simulink model "plant898708"  (R2016b)
settings: Solver=VariableStepAuto  StartTime=0.0  StopTime=800  RelTol=0.6
InitFcn:
  | data898708
undefined symbols (not defined in the file): En, ien, J, Keq, ki_ie, ki_ome, kp_ia, kp_ie, kp_ome, kr, La, Le, M, ome_n, r, Ra, Re, Ti_ia, Ti_ie, Ti_ome
settings Model: Creator=caidomenico  LastModifiedBy=caidomenico
settings SolverCC: ZeroCrossAlgorithm=Adaptive

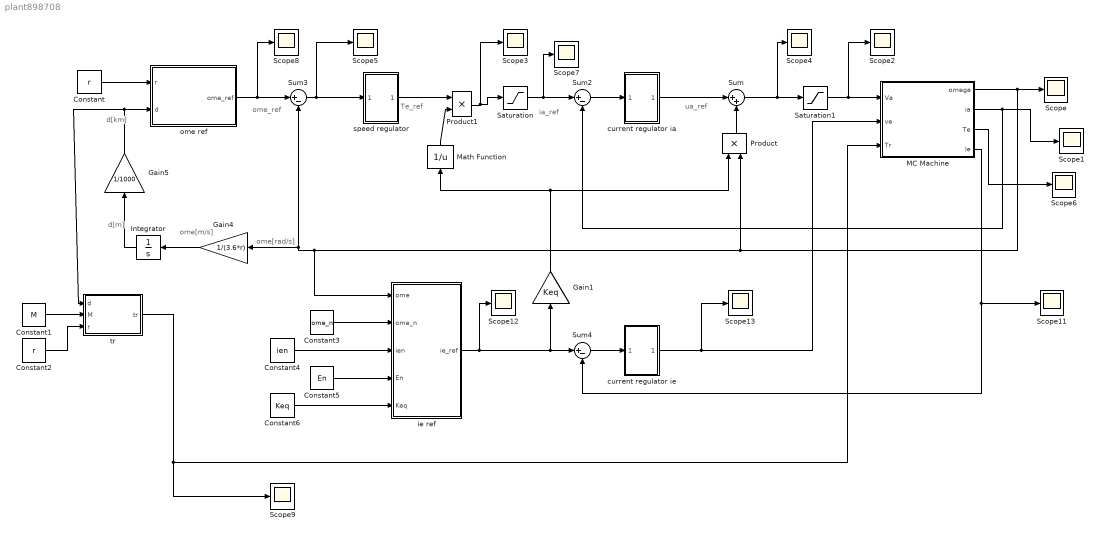
== system plant898708 ==
  note: ua_ref
  note: ia_ref
  note: Te_ref
  note: ome_ref
  note: d[km]
  note: d[m]
  note: ome[rad/s]
  note: ome[m/s]
  Constant : Constant  Value=r
  Constant1 : Constant  Value=M
  Constant2 : Constant  Value=r
  Constant3 : Constant  Value=ome_n
  Constant4 : Constant  Value=ien
  Constant5 : Constant  Value=En
  Constant6 : Constant  Value=Keq
  Gain1 : Gain  Gain=Keq
  Gain4 : Gain  Gain=1/(3.6*r)
  Gain5 : Gain  Gain=1/1000
  Integrator : Integrator
  MC Machine : Subsystem
      mask DialogControl DescTextVar Prompt: %<DC>
  Math Function : Math  Operator=reciprocal  SaturateOnIntegerOverflow=on
  Product : Product
  Product1 : Product
  Saturation : Saturate  UpperLimit=713  LowerLimit=0
  Saturation1 : Saturate  UpperLimit=600
  Scope{,1..9,11..13} (13 alike) : Scope
  Sum : Sum  Inputs=|++
  Sum2 : Sum  Inputs=|+-
  Sum3 : Sum  Inputs=|+-
  Sum4 : Sum  Inputs=|+-
  current regulator ia : Subsystem
  current regulator ie : Subsystem
  ie ref : MATLAB Function  TreatAsAtomicUnit=on
  ome ref : MATLAB Function  TreatAsAtomicUnit=on
  speed regulator : Subsystem
  tr : MATLAB Function  TreatAsAtomicUnit=on
  wires:
  Sum3/1 -> speed regulator/1(In1), Scope5/1
  MC Machine/1(omega) -> Product/2, ie ref/1(ome), Sum3/2, Gain4/1, Scope/1
  MC Machine/2(ia) -> Sum2/2, Scope1/1
  Sum/1 -> Scope4/1, Saturation1/1
  Saturation1/1 -> Scope2/1, MC Machine/1(Va)
  MC Machine/3(Te) -> Scope6/1
  ome ref/1(ome_ref) -> Scope8/1, Sum3/1
  Gain4/1 -> Integrator/1
  Integrator/1 -> Gain5/1
  Gain5/1 -> tr/1(d), ome ref/2(d)
  Constant/1 -> ome ref/1(r)
  speed regulator/1(Out1) -> Product1/1
  Constant3/1 -> ie ref/2(ome_n)
  Constant4/1 -> ie ref/3(ien)
  Constant5/1 -> ie ref/4(En)
  Constant6/1 -> ie ref/5(Keq)
  ie ref/1(ie_ref) -> Sum4/1, Gain1/1, Scope12/1
  Sum4/1 -> current regulator ie/1(In1)
  MC Machine/4(le) -> Scope11/1, Sum4/2
  current regulator ie/1(Out1) -> Scope13/1, MC Machine/2(ve)
  Sum2/1 -> current regulator ia/1(In1)
  current regulator ia/1(Out1) -> Sum/1
  Product1/1 -> Saturation/1, Scope3/1
  Product/1 -> Sum/2
  Gain1/1 -> Product/1, Math Function/1
  Math Function/1 -> Product1/2
  Saturation/1 -> Scope7/1, Sum2/1
  Constant1/1 -> tr/2(M)
  tr/1(tr) -> Scope9/1, MC Machine/3(Tr)
  Constant2/1 -> tr/3(r)

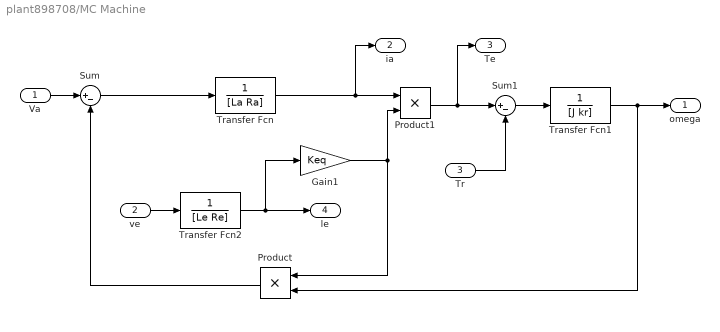
== system plant898708/MC Machine ==
  Va : Inport
  ve : Inport  Port=2
  Tr : Inport  Port=3
  Gain1 : Gain  Gain=Keq
  Product : Product
  Product1 : Product
  Sum : Sum  Inputs=|+-
  Sum1 : Sum  Inputs=|+-
  Transfer Fcn : TransferFcn  Denominator=[La Ra]
  Transfer Fcn1 : TransferFcn  Denominator=[J kr]
  Transfer Fcn2 : TransferFcn  Denominator=[Le Re]
  omega : Outport
  ia : Outport  Port=2
  Te : Outport  Port=3
  le : Outport  Port=4
  wires:
  Va/1 -> Sum/1
  Transfer Fcn/1 -> Product1/1, ia/1
  Sum/1 -> Transfer Fcn/1
  Transfer Fcn1/1 -> omega/1, Product/2
  ve/1 -> Transfer Fcn2/1
  Transfer Fcn2/1 -> le/1, Gain1/1
  Product1/1 -> Te/1, Sum1/1
  Gain1/1 -> Product/1, Product1/2
  Product/1 -> Sum/2
  Tr/1 -> Sum1/2
  Sum1/1 -> Transfer Fcn1/1

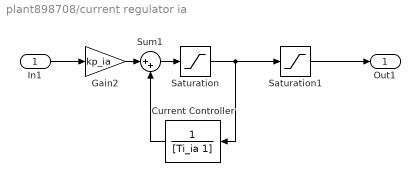
== system plant898708/current regulator ia ==
  In1 : Inport
  Current Controller : TransferFcn  Denominator=[Ti_ia 1]
  Gain2 : Gain  Gain=kp_ia
  Saturation : Saturate  UpperLimit=600
  Saturation1 : Saturate  UpperLimit=600
  Sum1 : Sum  Inputs=|++
  Out1 : Outport
  wires:
  Gain2/1 -> Sum1/1
  In1/1 -> Gain2/1
  Current Controller/1 -> Sum1/2
  Sum1/1 -> Saturation/1
  Saturation/1 -> Saturation1/1, Current Controller/1
  Saturation1/1 -> Out1/1

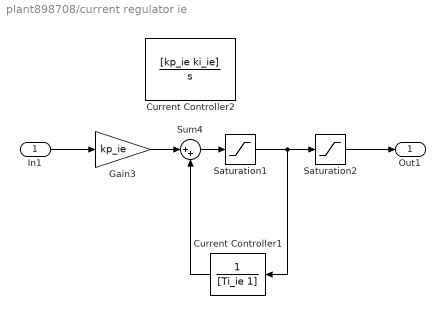
== system plant898708/current regulator ie ==
  In1 : Inport
  Current Controller1 : TransferFcn  Denominator=[Ti_ie 1]
  Current Controller2 : TransferFcn  Numerator=[kp_ie ki_ie]  Denominator=[1 0]
  Gain3 : Gain  Gain=kp_ie
  Saturation1 : Saturate  UpperLimit=120  LowerLimit=0
  Saturation2 : Saturate  UpperLimit=120  LowerLimit=0
  Sum4 : Sum  Inputs=|++
  Out1 : Outport
  wires:
  Current Controller1/1 -> Sum4/2
  Saturation1/1 -> Saturation2/1, Current Controller1/1
  Gain3/1 -> Sum4/1
  Sum4/1 -> Saturation1/1
  In1/1 -> Gain3/1
  Saturation2/1 -> Out1/1

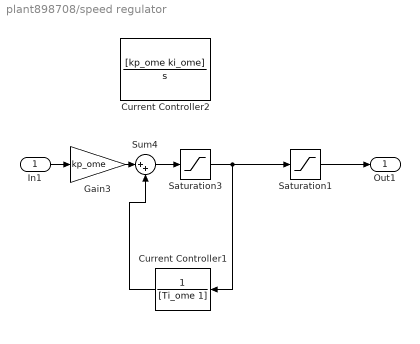
== system plant898708/speed regulator ==
  In1 : Inport
  Current Controller1 : TransferFcn  Denominator=[Ti_ome 1]
  Current Controller2 : TransferFcn  Numerator=[kp_ome ki_ome]  Denominator=[1 0]
  Gain3 : Gain  Gain=kp_ome
  Saturation1 : Saturate  UpperLimit=713*Keq  LowerLimit=0
  Saturation3 : Saturate  UpperLimit=713*Keq  LowerLimit=0
  Sum4 : Sum  Inputs=|++
  Out1 : Outport
  wires:
  Current Controller1/1 -> Sum4/2
  Saturation3/1 -> Saturation1/1, Current Controller1/1
  Gain3/1 -> Sum4/1
  Sum4/1 -> Saturation3/1
  In1/1 -> Gain3/1
  Saturation1/1 -> Out1/1

== matlab function plant898708/ie ref ==
  data: ome input; ie_ref output; ome_n input; ien input; En input; Keq input
function ie_ref = fcn(ome,ome_n,ien,En,Keq)
if ome<=ome_n
    ie_ref=ien;
else
    ie_ref=En/(Keq*ome);
end

== matlab function plant898708/ome ref ==
  data: r input; d input; ome_ref output
function ome_ref = fcn(r,d)
if d<=1
    ome_ref=r*35;
elseif d>1 && d<=4
    ome_ref=r*60;
elseif d>4 && d<=6
    ome_ref=r*75;
elseif d>6 && d<=9
    ome_ref=r*60;
elseif d>9 && d<=10
    ome_ref=r*35;
else 
    ome_ref=0;
end

== matlab function plant898708/tr ==
  data: d input; tr output; M input; r input
function tr = fcn(d,M,r)
if d>3 && d<=4
    tr=M*9.8*0.0005/r;
elseif d>8 && d<=9
    tr=-M*9.8*0.0005/r;
else
    tr=0;
end
